simulink model "simulace_odezev"  (R2015b)
settings: Solver=VariableStepAuto  StartTime=0.0  StopTime=10  RelTol=1e-3
values from neighbouring files (symbols this model uses):
  alpha = n * Kt / Rm    (= 0.0473841554559)    [parametry_segwaye_moje_upravene.m]
  beta = n * Kt * Kb / Rm + fm    (= 0.0243757847534)    [parametry_segwaye_moje_upravene.m]
  fw = 0    [parametry_segwaye_moje_upravene.m]
  g = 9.81    [parametry_segwaye_moje_upravene.m]
  Jm = 1e-5    (= 1e-05)    [parametry_segwaye_moje_upravene.m]
  Jpsi = M * L^2 / 3    (= 0.00123733333333)    [parametry_segwaye_moje_upravene.m]
  Jw = m * R^2 / 2    (= 2.4e-05)    [parametry_segwaye_moje_upravene.m]
  L = H / 2    (= 0.08)    [parametry_segwaye_moje_upravene.m]
  m = 0.03    [parametry_segwaye_moje_upravene.m]
  M = 0.58    [parametry_segwaye_moje_upravene.m]
  maticeA = [0 0 1 0; 0 0 0 1; 0 a(3) a(2) a(1); 0 a(7) a(6) a(5)]    [parametry_segwaye_moje_upravene.m]
  maticeB = [0; 0; a(4); a(8)]    [parametry_segwaye_moje_upravene.m]
  n = 1    [parametry_segwaye_moje_upravene.m]
  R = 0.04    [parametry_segwaye_moje_upravene.m]
  stavova_ZV = acker(maticeA, maticeB, desired_poles)    [navrh_stavove_zpetne_vazby.m]
libraries: simulink x1
settings Model: Creator=Já  LastModifiedBy=Já

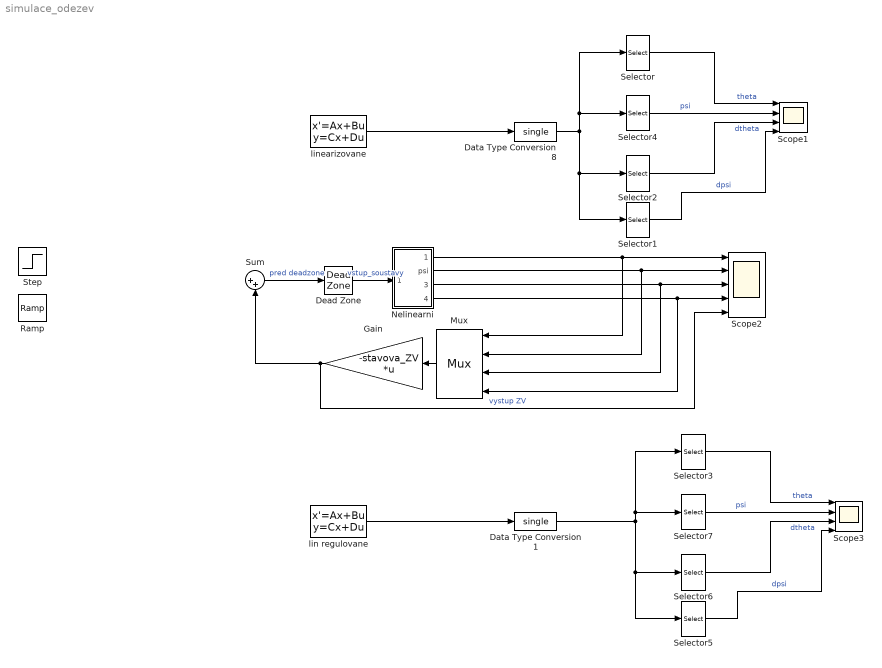
== system simulace_odezev ==
  Data Type Conversion1 : DataTypeConversion  OutDataTypeStr=single  RndMeth=Nearest
  Data Type Conversion8 : DataTypeConversion  OutDataTypeStr=single  RndMeth=Nearest
  Dead Zone : DeadZone  LowerValue=-0.22  UpperValue=0.3  SaturateOnIntegerOverflow=on
  Gain : Gain  Gain=-stavova_ZV  Multiplication=Matrix(K*u)
  Mux : Mux
      settings: DisplayOption=signals
  "Nelinearni " : Subsystem
  Ramp : simulink/Sources/Ramp  slope=1  start=0  X0=0
  Scope1 : Scope  NumInputPorts=4
  Scope2 : Scope  NumInputPorts=5
  Scope3 : Scope  NumInputPorts=4
  Selector : Selector  InputPortWidth=4  IndexOptions=Index vector (dialog)  Indices=1  OutputSizes=1
  Selector1 : Selector  InputPortWidth=4  IndexOptions=Index vector (dialog)  Indices=4  OutputSizes=1
  Selector2 : Selector  InputPortWidth=4  IndexOptions=Index vector (dialog)  Indices=3  OutputSizes=1
  Selector3 : Selector  InputPortWidth=4  IndexOptions=Index vector (dialog)  Indices=1  OutputSizes=1
  Selector4 : Selector  InputPortWidth=4  IndexOptions=Index vector (dialog)  Indices=2  OutputSizes=1
  Selector5 : Selector  InputPortWidth=4  IndexOptions=Index vector (dialog)  Indices=4  OutputSizes=1
  Selector6 : Selector  InputPortWidth=4  IndexOptions=Index vector (dialog)  Indices=3  OutputSizes=1
  Selector7 : Selector  InputPortWidth=4  IndexOptions=Index vector (dialog)  Indices=2  OutputSizes=1
  Step : Step  After=0  SampleTime=0
  Sum : Sum  Inputs=|++
  lin regulovane : StateSpace  A=maticeA - maticeB*stavova_ZV  B=maticeB  C=eye(4)  D=zeros(4,1)  X0=zeros(4,1)
  linearizovane : StateSpace  A=maticeA  B=maticeB  C=eye(4)  D=zeros(4,1)  X0=zeros(4,1)
  wires:
  Data Type Conversion8/1 -> Selector/1, Selector4/1, Selector2/1, Selector1/1
  Selector1/1 -> Scope1/4  "dpsi"
  Selector/1 -> Scope1/1  "theta"
  Selector4/1 -> Scope1/2  "psi"
  Selector2/1 -> Scope1/3  "dtheta"
  linearizovane/1 -> Data Type Conversion8/1
  ? -> Sum/1, linearizovane/1, lin regulovane/1
  "Nelinearni "/1(theta) -> Mux/1, Scope2/1
  "Nelinearni "/3(theta dot) -> Mux/3, Scope2/3
  "Nelinearni "/4(psi dot) -> Mux/4, Scope2/4
  Data Type Conversion1/1 -> Selector5/1, Selector6/1, Selector3/1, Selector7/1
  Selector5/1 -> Scope3/4  "dpsi"
  Selector3/1 -> Scope3/1  "theta"
  Selector7/1 -> Scope3/2  "psi"
  Selector6/1 -> Scope3/3  "dtheta"
  lin regulovane/1 -> Data Type Conversion1/1
  Mux/1 -> Gain/1
  Sum/1 -> Dead Zone/1  "pred deadzone"
  Dead Zone/1 -> "Nelinearni "/1(voltage)  "vstup_soustavy"
  Gain/1 -> Sum/2, Scope2/5  "vystup ZV"
  "Nelinearni "/2(psi) -> Mux/2, Scope2/2

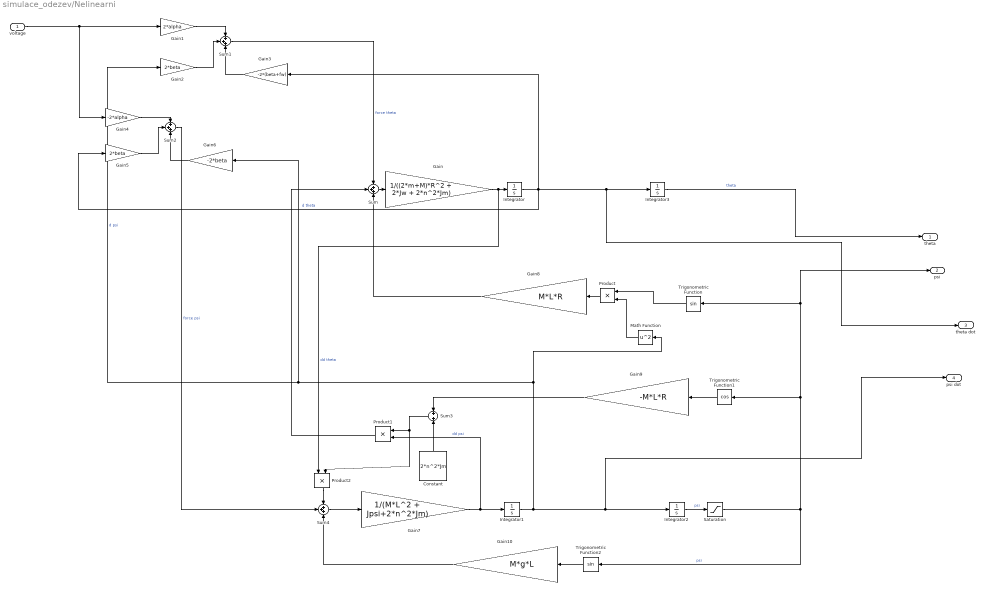
== system simulace_odezev/Nelinearni  ==
  voltage : Inport
  Constant : Constant  Value=2*n^2*Jm
  Gain : Gain  Gain=1/((2*m+M)*R^2 + 2*Jw + 2*n^2*Jm)
  Gain1 : Gain  Gain=2*alpha
  Gain10 : Gain  Gain=M*g*L
  Gain2 : Gain  Gain=2*beta
  Gain3 : Gain  Gain=-2*(beta+fw)
  Gain4 : Gain  Gain=-2*alpha
  Gain5 : Gain  Gain=2*beta
  Gain6 : Gain  Gain=-2*beta
  Gain7 : Gain  Gain=1/(M*L^2 + Jpsi+2*n^2*Jm)
  Gain8 : Gain  Gain=M*L*R
  Gain9 : Gain  Gain=-M*L*R
  Integrator : Integrator
  Integrator1 : Integrator
  Integrator2 : Integrator  InitialCondition=pi/12
  Integrator3 : Integrator
  Math Function : Math  Operator=square  SaturateOnIntegerOverflow=on
  Product : Product
  Product1 : Product
  Product2 : Product
  Saturation : Saturate  UpperLimit=pi/2  LowerLimit=-pi/2
  Sum{,1..2,4} (4 alike) : Sum  Inputs=+++
  Sum3 : Sum
  Trigonometric Function : Trigonometry
  Trigonometric Function1 : Trigonometry  Operator=cos
  Trigonometric Function2 : Trigonometry
  theta : Outport
  psi : Outport  Port=2
  theta dot : Outport  Port=3
  psi dot : Outport  Port=4
  wires:
  Gain/1 -> Product2/1, Integrator/1  "dd theta"
  Integrator1/1 -> Math Function/1, Gain6/1, Gain2/1, psi dot/1, Integrator2/1  "d psi"
  Integrator/1 -> Gain5/1, Gain3/1, theta dot/1, Integrator3/1  "d theta"
  Gain7/1 -> Product1/2, Integrator1/1  "dd psi"
  Sum/1 -> Gain/1
  Trigonometric Function/1 -> Product/1
  Product/1 -> Gain8/1
  Constant/1 -> Sum3/2
  Gain2/1 -> Sum1/2
  Gain3/1 -> Sum1/3
  Product1/1 -> Sum/2
  Gain9/1 -> Sum3/1
  Gain1/1 -> Sum1/1
  voltage/1 -> Gain4/1, Gain1/1
  Gain8/1 -> Sum/3
  Sum3/1 -> Product2/2, Product1/1
  Sum1/1 -> Sum/1  "force theta"
  Gain6/1 -> Sum2/3
  Math Function/1 -> Product/2
  Gain5/1 -> Sum2/2
  Gain4/1 -> Sum2/1
  Product2/1 -> Sum4/1
  Gain10/1 -> Sum4/3
  Trigonometric Function2/1 -> Gain10/1
  Sum4/1 -> Gain7/1
  Sum2/1 -> Sum4/2  "force psi"
  Trigonometric Function1/1 -> Gain9/1
  Saturation/1 -> Trigonometric Function2/1, psi/1, Trigonometric Function/1, Trigonometric Function1/1  "psi"
  Integrator2/1 -> Saturation/1  "psi"
  Integrator3/1 -> theta/1  "theta"
